simulink model "day5"  (R2025b)
settings: Solver=VariableStepAuto  StartTime=0.0  StopTime=20  RelTol=1e-3
undefined symbols (not defined in the file or in its folder): K01, omega01, T01, zeta01
settings Model: Creator=tumik  LastModifiedBy=tumik

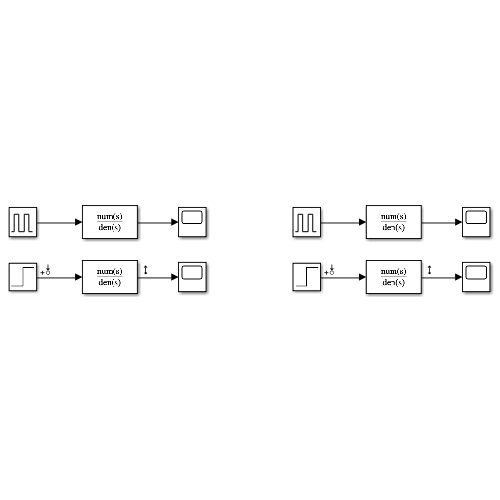
[thumbnail: Simulink's stored preview of the top-level diagram]
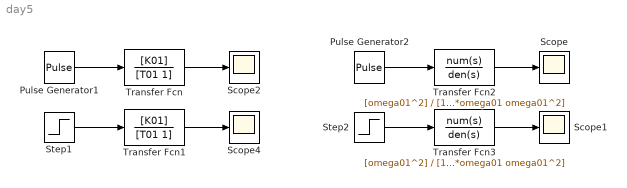
== system day5 ==
  Pulse Generator1 : DiscretePulseGenerator  PulseType=Time based  Amplitude=500  Period=20  PulseWidth=0.01  PhaseDelay=1
  Pulse Generator2 : DiscretePulseGenerator  PulseType=Time based  Amplitude=500  Period=20  PulseWidth=0.01  PhaseDelay=1
  Scope{,1..2,4} (4 alike) : Scope
      Scope settings: ActiveDisplayYMinimum=-1  ActiveDisplayYMaximum=1
      Scope1 settings: ActiveDisplayYMinimum=-1  ActiveDisplayYMaximum=1
      Scope2 settings: ActiveDisplayYMinimum=-1  ActiveDisplayYMaximum=1  DataLoggingVariableName=ScopeData2
      Scope4 settings: ActiveDisplayYMinimum=-0.10639012780936774  ActiveDisplayYMaximum=2.0967121553543988  DataLoggingVariableName=ScopeData4
  Step1 : Step  SampleTime=0
  Step2 : Step  SampleTime=0
  Transfer Fcn : TransferFcn  Numerator=[K01]  Denominator=[T01 1]
  Transfer Fcn1 : TransferFcn  Numerator=[K01]  Denominator=[T01 1]
  Transfer Fcn2 : TransferFcn  Numerator=[omega01^2]  Denominator=[1 2*zeta01*omega01 omega01^2]
  Transfer Fcn3 : TransferFcn  Numerator=[omega01^2]  Denominator=[1 2*zeta01*omega01 omega01^2]
  wires:
  Pulse Generator1/1 -> Transfer Fcn/1
  Step1/1 -> Transfer Fcn1/1
  Pulse Generator2/1 -> Transfer Fcn2/1
  Step2/1 -> Transfer Fcn3/1
  Transfer Fcn/1 -> Scope2/1
  Transfer Fcn1/1 -> Scope4/1
  Transfer Fcn2/1 -> Scope/1
  Transfer Fcn3/1 -> Scope1/1
